simulink model "Force2Axis"  (R2022b)
settings: configuration reference "WheelSimConfiguration" (kept outside this file)
undefined symbols (not defined in the file): simulator
settings Model: SimulationMode=external  Creator=At  LastModifiedBy=MOSA
settings ConfigSetRef: SourceName=WheelSimConfiguration  SourceLocation=Base Workspace

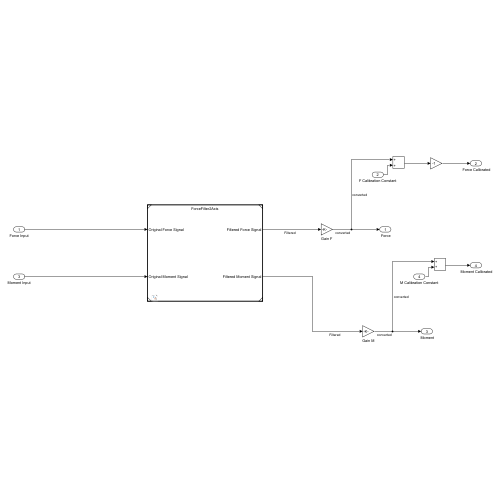
[thumbnail: Simulink's stored preview of the top-level diagram]
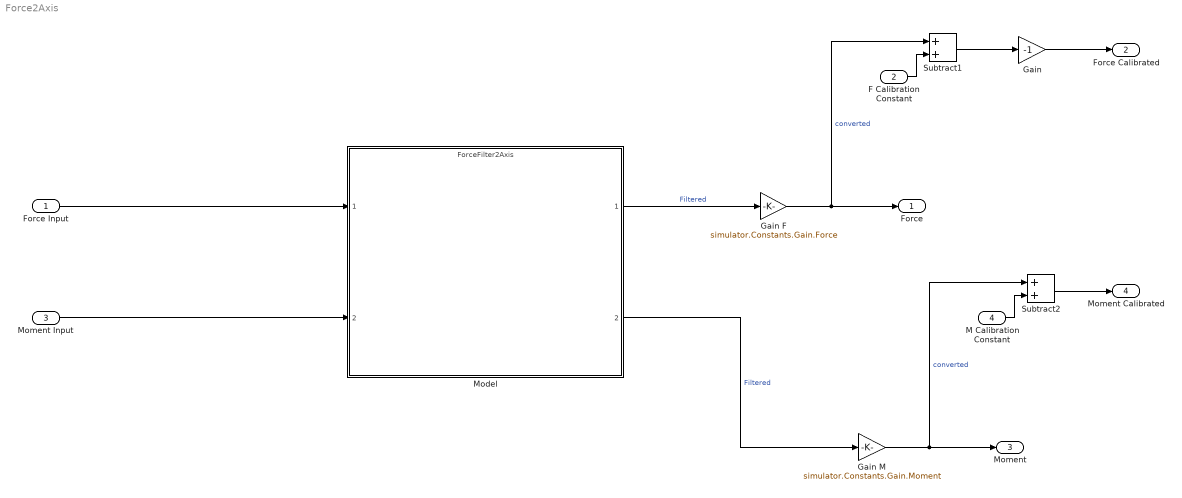
== system Force2Axis ==
  Force Input : Inport
  F Calibration Constant : Inport  Port=2
  Moment Input : Inport  Port=3
  M Calibration Constant : Inport  Port=4
  Gain : Gain  Gain=-1
  Gain F : Gain  Gain=simulator.Constants.Gain.Force
  Gain M : Gain  Gain=simulator.Constants.Gain.Moment
  Model : ModelReference  ModelNameDialog=ForceFilter2Axis.slx  SimulationMode=Normal  ModelReferenceVersion=13.4
  Subtract1 : Sum
  Subtract2 : Sum
  " Force" : Outport
  " Force Calibrated" : Outport  Port=2
  " Moment" : Outport  Port=3
  " Moment Calibrated" : Outport  Port=4
  wires:
  Force Input/1 -> Model/1
  Model/1 -> Gain F/1  "Filtered"
  F Calibration Constant/1 -> Subtract1/2
  Gain F/1 -> " Force"/1, Subtract1/1  "converted"
  Subtract1/1 -> Gain/1
  Moment Input/1 -> Model/2
  Gain M/1 -> " Moment"/1, Subtract2/1  "converted"
  M Calibration Constant/1 -> Subtract2/2
  Subtract2/1 -> " Moment Calibrated"/1
  Model/2 -> Gain M/1  "Filtered"
  Gain/1 -> " Force Calibrated"/1
